simulink model "ncmexample"  (R2012a)
settings: Solver=ode3  StartTime=0.0  StopTime=10.0  FixedStep=0.125  RelTol=1e-3
libraries: truetime x7, NCM x1
settings Model: ExtModeAutoUpdateStatusClock=off  Creator=sf  LastModifiedBy=anton
settings DataIOCC: LimitDataPoints=on  SaveFormat=Array  SignalLoggingSaveFormat=ModelDataLogs  ReturnWorkspaceOutputs=off
settings OptimizationCC: ExpressionDepthLimit=2147483647  InitFltsAndDblsToZero=on  LifeSpan=inf  SimCompilerOptimization=Off
settings DebuggingCC: SaveWithParameterizedLinksMsg=none  UnderspecifiedInitializationDetection=Classic  MergeDetectMultiDrivingBlocksExec=none  SolverPrmCheckMsg=warning  FcnCallInpInsideContextMsg=Use local settings  StateNameClashWarn=warning  StrictBusMsg=Warning  SFUnexpectedBacktrackingDiag=warning  SFNoUnconditionalDefaultTransitionDiag=warning
settings HardwareCC: ProdBitPerPointer=32  ProdLargestAtomicFloat=None  ProdIntDivRoundTo=Undefined  ProdEndianess=Unspecified  ProdWordSize=32  ProdHWDeviceType=32-bit Generic
settings ModelReferenceCC: PropagateSignalLabelsOutOfModel=off
settings SFSimCC: SimUseLocalCustomCode=off  SimParseCustomCode=off
settings RTWCC: RTWUseLocalCustomCode=off  RTWCompilerOptimization=Off
settings GRTTargetCC: TargetFcnLib=ansi_tfl_tmw.mat  CodeReplacementLibrary=C89/C90 (ANSI)  GeneratePreprocessorConditionals=Disable all  CombineOutputUpdateFcns=off  CPPClassGenCompliant=off  GRTInterface=on

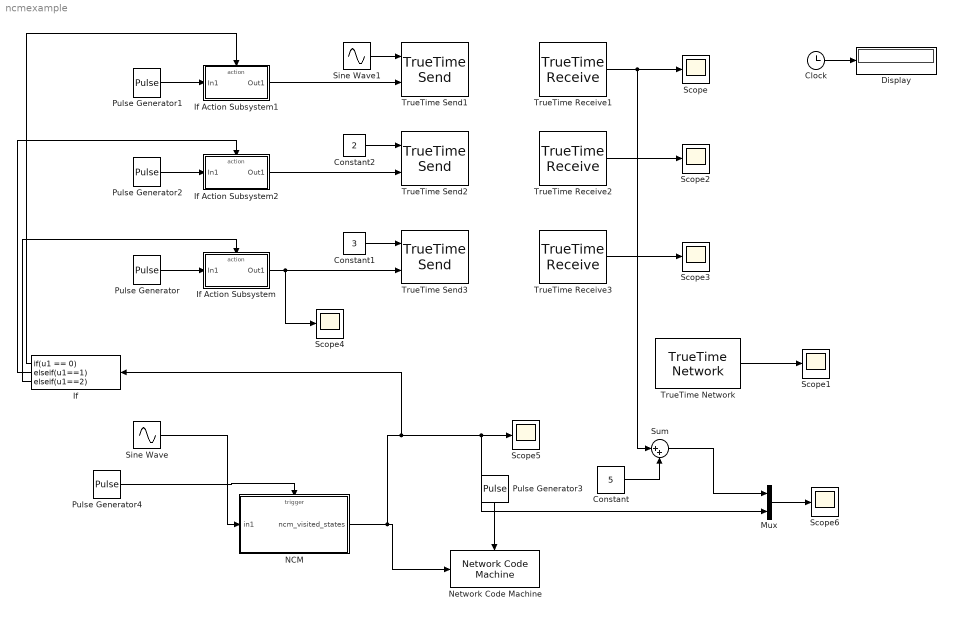
== system ncmexample ==
  Clock : Clock
  Constant : Constant  Value=5
  Constant1 : Constant  Value=3
  Constant2 : Constant  Value=2
  Display : Display
  If : If  IfExpression=u1 == 0  ElseIfExpressions=u1==1,u1==2  ShowElse=off
  If Action Subsystem : Subsystem  TreatAsAtomicUnit=on
  If Action Subsystem1 : Subsystem  TreatAsAtomicUnit=on
  If Action Subsystem2 : Subsystem  TreatAsAtomicUnit=on
  Mux : Mux  Inputs=2
  NCM : Stateflow chart  TreatAsAtomicUnit=on
      settings: PermitHierarchicalResolution=ParametersOnly
  Network Code Machine : NCM/Network Code Machine
  Pulse Generator : DiscretePulseGenerator  PulseType=Time based  Period=0.5  PulseWidth=50
  Pulse Generator1 : DiscretePulseGenerator  PulseType=Time based  Period=0.5  PulseWidth=50
  Pulse Generator2 : DiscretePulseGenerator  PulseType=Time based  Period=0.5  PulseWidth=50
  Pulse Generator3 : DiscretePulseGenerator  PulseType=Time based  Period=0.25  PulseWidth=50  PhaseDelay=.5
  Pulse Generator4 : DiscretePulseGenerator  PulseType=Time based  Period=0.25  PulseWidth=50
  Scope{,1..6} (7 alike) : Scope
      Scope settings: TimeRange=auto  LimitDataPoints=on  MaxDataPoints=5000  SaveToWorkspace=off  SaveName=ScopeData  YMin=0  YMax=3  SampleTime=-1
      Scope1 settings: TimeRange=auto  LimitDataPoints=on  MaxDataPoints=5000  SaveToWorkspace=off  YMin=0.6875  YMax=3.8125  SampleTime=-1
      Scope2 settings: TimeRange=auto  LimitDataPoints=on  MaxDataPoints=5000  SaveToWorkspace=off  SaveName=ScopeData2  YMin=-10  YMax=10  SampleTime=-1
      Scope3 settings: TimeRange=auto  LimitDataPoints=on  MaxDataPoints=5000  SaveToWorkspace=off  SaveName=ScopeData3  YMin=-10  YMax=10  SampleTime=-1
      Scope4 settings: TimeRange=auto  LimitDataPoints=on  MaxDataPoints=5000  SaveToWorkspace=off  SaveName=ScopeData4  YMin=-10  YMax=10  SampleTime=-1
      Scope5 settings: TimeRange=auto  LimitDataPoints=on  MaxDataPoints=5000  SaveToWorkspace=off  SaveName=ScopeData5  YMin=-10  YMax=10  SampleTime=-1
      Scope6 settings: TimeRange=auto  LimitDataPoints=on  MaxDataPoints=5000  SaveToWorkspace=off  SaveName=ScopeData6  YMin=0  YMax=3  SampleTime=-1
  Sine Wave : Sin  SampleTime=0
  Sine Wave1 : Sin  SampleTime=0
  Sum : Sum  Inputs=|++
  TrueTime Network : truetime/TrueTime Network  nwtype=NCM  nwnbr=1  nnodes=3  rate=10000000  minsize=512  lossprob=0  seed=0  bandwidths=[0.5 0.5]  slotsize=512  schedule=[1 1 2]  memsize=80000  buftype=Common buffer  overflow=Retransmit  dynSchedule=0  miniSlotSize=0  NIT=0  QSortMode=FIFO  sync=0  irtSchedule=0  nrtLength=0  nodeGraph=0  scheduleoutput=on
  TrueTime Receive1 : truetime/TrueTime Receive  nwnbr=1  receiver=1  outdim=1  triggeroutput=off  senderoutput=off  lengthoutput=off  priorityoutput=off  timestampoutput=off  signalpoweroutput=off  msgIDoutput=off
  TrueTime Receive2 : truetime/TrueTime Receive  nwnbr=1  receiver=2  outdim=1  triggeroutput=off  senderoutput=off  lengthoutput=off  priorityoutput=off  timestampoutput=off  signalpoweroutput=off  msgIDoutput=off
  TrueTime Receive3 : truetime/TrueTime Receive  nwnbr=1  receiver=3  outdim=1  triggeroutput=off  senderoutput=off  lengthoutput=off  priorityoutput=off  timestampoutput=off  signalpoweroutput=off  msgIDoutput=off
  TrueTime Send1 : truetime/TrueTime Send  trigger=falling  nwnbr=1  sender=1  indim=1  recsource=internal  receiver=1  lengthsource=internal  length=1000  priosource=internal  prio=1  msgIDsource=internal  msgID=0  dynamicSegment=dynamic
  TrueTime Send2 : truetime/TrueTime Send  trigger=falling  nwnbr=1  sender=2  indim=1  recsource=internal  receiver=1  lengthsource=internal  length=1000  priosource=internal  prio=1  msgIDsource=internal  msgID=0  dynamicSegment=dynamic
  TrueTime Send3 : truetime/TrueTime Send  trigger=falling  nwnbr=1  sender=3  indim=1  recsource=internal  receiver=1  lengthsource=internal  length=1000  priosource=internal  prio=1  msgIDsource=internal  msgID=0  dynamicSegment=dynamic
  wires:
  Clock/1 -> Display/1
  TrueTime Network/1 -> Scope1/1
  Pulse Generator3/1 -> Network Code Machine/Trigger
  Sine Wave1/1 -> TrueTime Send1/1
  Constant1/1 -> TrueTime Send3/1
  Constant2/1 -> TrueTime Send2/1
  If/3 -> If Action Subsystem/Action
  If Action Subsystem/1(Out1) -> TrueTime Send3/2, Scope4/1
  If Action Subsystem2/1(Out1) -> TrueTime Send2/2
  If/2 -> If Action Subsystem2/Action
  If/1 -> If Action Subsystem1/Action
  If Action Subsystem1/1(Out1) -> TrueTime Send1/2
  Pulse Generator/1 -> If Action Subsystem/1(In1)
  Pulse Generator2/1 -> If Action Subsystem2/1(In1)
  Pulse Generator1/1 -> If Action Subsystem1/1(In1)
  TrueTime Receive1/1 -> Scope/1, Sum/1
  TrueTime Receive2/1 -> Scope2/1
  TrueTime Receive3/1 -> Scope3/1
  Pulse Generator4/1 -> NCM/Trigger
  NCM/1(ncm_visited_states) -> Network Code Machine/1, If/1, Scope5/1, Mux/2
  Sine Wave/1 -> NCM/1(in1)
  Mux/1 -> Scope6/1
  Constant/1 -> Sum/2
  Sum/1 -> Mux/1

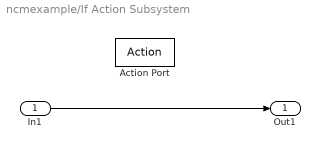
== system ncmexample/If Action Subsystem ==
  In1 : Inport
  Action Port : ActionPort  ActionType=elseif
  Out1 : Outport
  wires:
  In1/1 -> Out1/1

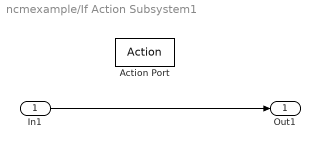
== system ncmexample/If Action Subsystem1 ==
  In1 : Inport
  Action Port : ActionPort  ActionType=then
  Out1 : Outport
  wires:
  In1/1 -> Out1/1

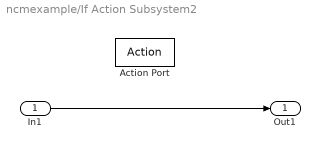
== system ncmexample/If Action Subsystem2 ==
  In1 : Inport
  Action Port : ActionPort  ActionType=elseif
  Out1 : Outport
  wires:
  In1/1 -> Out1/1

== stateflow chart ncmexample/NCM ==
  state NCM
    state node2
      entry: ncm_visited_states= 1;
    state node3
      entry:
      ncm_visited_states=2;
    state saved_state
      entry: ncm_visited_states=0;
    state node1
      entry: ncm_visited_states=0;
    node2 -> node3 [order 1] : after(1,CLOCK)...
        | [in1 > .5]
    node2 -> saved_state [order 2] : after(1,CLOCK)...
        | [ in1 <= .5]
    node1 -> node2 : after(1,CLOCK)...
    node3 -> node1 : after(1,CLOCK)...
    saved_state -> node1
    (default) -> node1
  data: ncm_visited_states output double; in1 input
  events: CLOCK input FALLING_EDGE_EVENT
